simulink model "sys10m_IO"  (Simulink 8.7)
settings: Solver=ode3  StartTime=0.0  StopTime=10  FixedStep=1e-2  MaxStep=1e-2  RelTol=1e-5
values from neighbouring files (symbols this model uses):
  D = 0*D    [initDyn.m]
  event = [0 1 1.10 10 ... (first row only)    [initDyn.m]
  fYred = fYGG-fYGL*inv(fYLL)*fYLG    [initDyn.m]
  KA = ExData(:,1)    [initDyn.m]
  M = 2*H/ws    [initDyn.m]
  m = 10    [initDyn.m]
  small_d = [ ... (first row only)    [initDyn.m]
  TA = ExData(:,2)    [initDyn.m]
  Tpd0 = GenData(:,6)    [initDyn.m]
  Tpq0 = GenData(:,7)    [initDyn.m]
  ws = 377    [initDyn.m]
  XXdpd = [Xd-Xpd]    [initDyn.m]
  XXpdq = [Xpq-Xpd]    [initDyn.m]
  XXqpq = [Xq-Xpq]    [initDyn.m]
  Yred = YGG-YGL*inv(YLL)*YLG    [initDyn.m]
  Zdq = [Rsm -Xpqm;Xpdm Rsm]    [initDyn.m]
undefined symbols (not defined in the file or in its folder): delta0, Efd0, Epd0, Epq0, Vref1
libraries: powerlib_extras x2
settings Model: Creator=hbeiran  LastModifiedBy=EBUKA
settings SolverCC: AlgebraicLoopSolver=LineSearch
settings DataIOCC: LimitDataPoints=off  SignalLoggingSaveFormat=ModelDataLogs
settings OptimizationCC: DefaultParameterBehavior=Inlined  BufferReuse=off  ExpressionDepthLimit=2147483647
settings DebuggingCC: AlgebraicLoopMsg=none  SolverPrmCheckMsg=warning  FcnCallInpInsideContextMsg=UseLocalSettings  StateNameClashWarn=warning  InitInArrayFormatMsg=none
settings SFSimCC: SimParseCustomCode=off
settings GRTTargetCC: CombineOutputUpdateFcns=off  GRTInterface=on

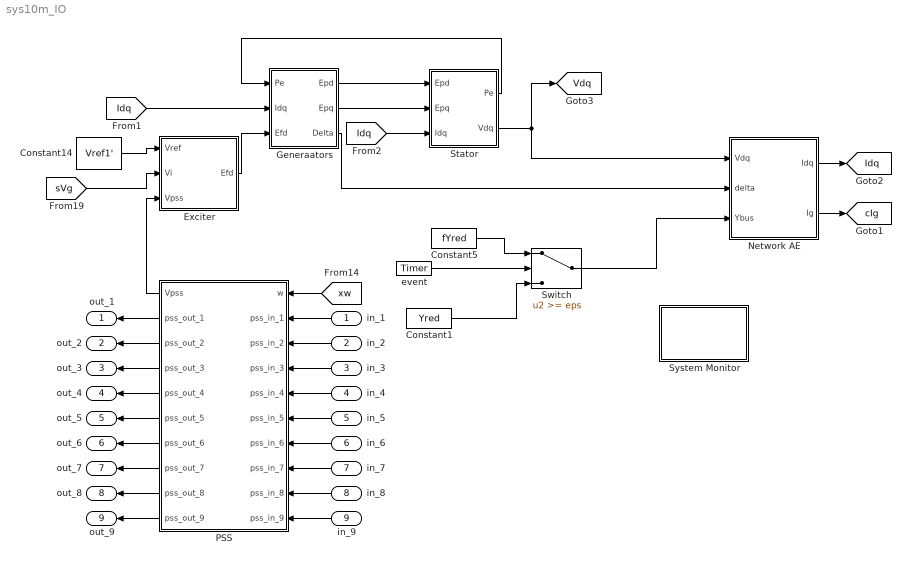
== system sys10m_IO ==
  in_1 : Inport
  in_2 : Inport  Port=2
  in_3 : Inport  Port=3
  in_4 : Inport  Port=4
  in_5 : Inport  Port=5
  in_6 : Inport  Port=6
  in_7 : Inport  Port=7
  in_8 : Inport  Port=8
  in_9 : Inport  Port=9
  Constant1 : Constant  Value=Yred  VectorParams1D=off
  Constant14 : Constant  Value=Vref1'  VectorParams1D=off
  Constant5 : Constant  Value=fYred  VectorParams1D=off
  Exciter : Subsystem
  Generaators : Subsystem
  Network AE : MATLAB Function  TreatAsAtomicUnit=on
  PSS : Subsystem
  Stator : Subsystem
  Switch : Switch  Threshold=eps
  System Monitor : Subsystem
  event : powerlib_extras/Control  Blocks/Timer  t=event(1,:)  e=event(2,:)
  out_1 : Outport
  out_2 : Outport  Port=2
  out_3 : Outport  Port=3
  out_4 : Outport  Port=4
  out_5 : Outport  Port=5
  out_6 : Outport  Port=6
  out_7 : Outport  Port=7
  out_8 : Outport  Port=8
  out_9 : Outport  Port=9
  tag scope: Idq=global, Vdq=global, cIg=global
  wires:
  Exciter/1(Efd) -> Generaators/3(Efd)
  Constant14/1 -> Exciter/1(Vref)
  Network AE/1(Idq) -> [Idq]
  event/1 -> Switch/2
  Constant5/1 -> Switch/1
  Constant1/1 -> Switch/3
  Switch/1 -> Network AE/3(Ybus)
  Generaators/3(Delta) -> Network AE/2(delta)
  Network AE/2(Ig) -> [cIg]
  Stator/2(Vdq) -> [Vdq], Network AE/1(Vdq)
  [Idq] -> Stator/3(Idq)
  Generaators/1(Epd) -> Stator/1(Epd)
  Generaators/2(Epq) -> Stator/2(Epq)
  Stator/1(Pe) -> Generaators/1(Pe)
  [sVg] -> Exciter/2(Vi)
  [Idq] -> Generaators/2(Idq)
  [xw] -> PSS/1(w)
  in_1/1 -> PSS/2(pss_in_1)
  in_2/1 -> PSS/3(pss_in_2)
  PSS/1(Vpss) -> Exciter/3(Vpss)
  PSS/2(pss_out_1) -> out_1/1
  PSS/3(pss_out_2) -> out_2/1
  in_3/1 -> PSS/4(pss_in_3)
  in_4/1 -> PSS/5(pss_in_4)
  in_5/1 -> PSS/6(pss_in_5)
  in_6/1 -> PSS/7(pss_in_6)
  in_7/1 -> PSS/8(pss_in_7)
  in_8/1 -> PSS/9(pss_in_8)
  in_9/1 -> PSS/10(pss_in_9)
  PSS/4(pss_out_3) -> out_3/1
  PSS/5(pss_out_4) -> out_4/1
  PSS/6(pss_out_5) -> out_5/1
  PSS/7(pss_out_6) -> out_6/1
  PSS/8(pss_out_7) -> out_7/1
  PSS/9(pss_out_8) -> out_8/1
  PSS/10(pss_out_9) -> out_9/1

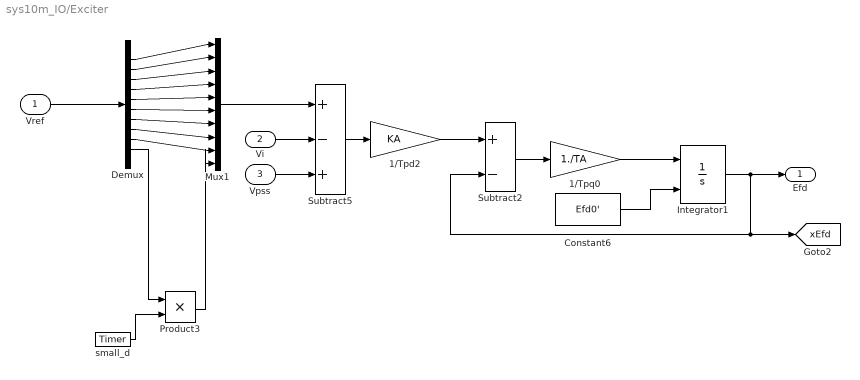
== system sys10m_IO/Exciter ==
  Vref : Inport
  Vi : Inport  Port=2
  Vpss : Inport  Port=3
  1/Tpd2 : Gain  Gain=KA
  1/Tpq0 : Gain  Gain=1./TA
  Constant6 : Constant  Value=Efd0'  VectorParams1D=off
  Demux : Demux  Outputs=10
  Integrator1 : Integrator  InitialConditionSource=external
  Mux1 : Mux  Inputs=10
  Product3 : Product  RndMeth=Zero
  Subtract2 : Sum  Inputs=+-
  Subtract5 : Sum  Inputs=+-+
  small_d : powerlib_extras/Control  Blocks/Timer  t=small_d(1,:)  e=small_d(2,:)
  Efd : Outport
  tag scope: xEfd=global
  wires:
  Constant6/1 -> Integrator1/2
  Subtract2/1 -> 1/Tpq0/1
  1/Tpq0/1 -> Integrator1/1
  Integrator1/1 -> Efd/1, Subtract2/2, [xEfd]
  Vi/1 -> Subtract5/2
  Subtract5/1 -> 1/Tpd2/1
  1/Tpd2/1 -> Subtract2/1
  Demux/1 -> Mux1/1
  Demux/2 -> Mux1/2
  small_d/1 -> Product3/2
  Mux1/1 -> Subtract5/1
  Vref/1 -> Demux/1
  Product3/1 -> Mux1/10
  Demux/10 -> Product3/1
  Demux/3 -> Mux1/3
  Demux/4 -> Mux1/4
  Demux/5 -> Mux1/5
  Demux/6 -> Mux1/6
  Demux/7 -> Mux1/7
  Demux/8 -> Mux1/8
  Demux/9 -> Mux1/9
  Vpss/1 -> Subtract5/3

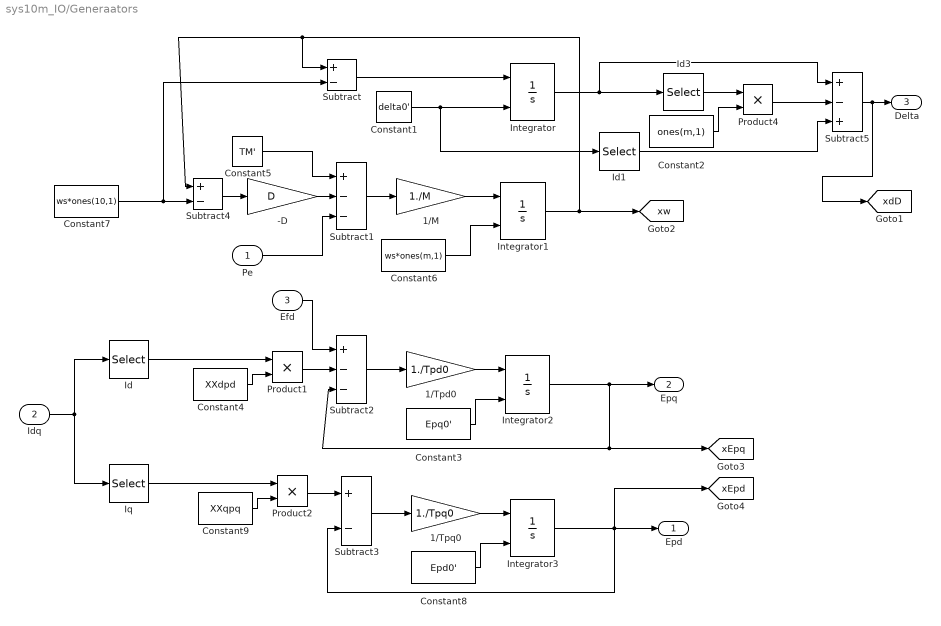
== system sys10m_IO/Generaators ==
  Pe : Inport
  Idq : Inport  Port=2
  Efd : Inport  Port=3
  -D : Gain  Gain=D
  1/M : Gain  Gain=1./M
  1/Tpd0 : Gain  Gain=1./Tpd0
  1/Tpq0 : Gain  Gain=1./Tpq0
  Constant1 : Constant  Value=delta0'  VectorParams1D=off
  Constant2 : Constant  Value=ones(m,1)  VectorParams1D=off
  Constant3 : Constant  Value=Epq0'  VectorParams1D=off
  Constant4 : Constant  Value=XXdpd  VectorParams1D=off
  Constant5 : Constant  Value=TM'  VectorParams1D=off
  Constant6 : Constant  Value=ws*ones(m,1)  VectorParams1D=off
  Constant7 : Constant  Value=ws*ones(10,1)  VectorParams1D=off
  Constant8 : Constant  Value=Epd0'  VectorParams1D=off
  Constant9 : Constant  Value=XXqpq  VectorParams1D=off
  Id : Selector  InputPortWidth=2*m  IndexOptions=Index vector (dialog)  Indices=[1:m]  OutputSizes=1
  Id1 : Selector  InputPortWidth=m  IndexOptions=Index vector (dialog)  Indices=[1]  OutputSizes=1
  Id3 : Selector  InputPortWidth=m  IndexOptions=Index vector (dialog)  Indices=[1]  OutputSizes=1
  Integrator{,1..3} (4 alike) : Integrator  InitialConditionSource=external
  Iq : Selector  InputPortWidth=2*m  IndexOptions=Index vector (dialog)  Indices=[m+1:2*m]  OutputSizes=1
  Product1 : Product  RndMeth=Zero
  Product2 : Product  RndMeth=Zero
  Product4 : Product  RndMeth=Zero
  Subtract : Sum  Inputs=+-
  Subtract1 : Sum  Inputs=+--
  Subtract2 : Sum  Inputs=+--
  Subtract3 : Sum  Inputs=+-
  Subtract4 : Sum  Inputs=+-
  Subtract5 : Sum  Inputs=+-+
  Epd : Outport
  Epq : Outport  Port=2
  Delta : Outport  Port=3
  tag scope: xEpd=global, xEpq=global, xdD=global, xw=global
  wires:
  Subtract/1 -> Integrator/1
  Constant5/1 -> Subtract1/1
  Subtract1/1 -> 1/M/1
  1/M/1 -> Integrator1/1
  Constant6/1 -> Integrator1/2
  -D/1 -> Subtract1/2
  Constant3/1 -> Integrator2/2
  Subtract2/1 -> 1/Tpd0/1
  Integrator2/1 -> Epq/1, Subtract2/3, [xEpq]
  Product1/1 -> Subtract2/2
  Constant4/1 -> Product1/2
  1/Tpd0/1 -> Integrator2/1
  Constant8/1 -> Integrator3/2
  Subtract3/1 -> 1/Tpq0/1
  Integrator3/1 -> Epd/1, [xEpd], Subtract3/2
  Constant9/1 -> Product2/2
  1/Tpq0/1 -> Integrator3/1
  Product2/1 -> Subtract3/1
  Efd/1 -> Subtract2/1
  Integrator1/1 -> [xw], Subtract/1, Subtract4/1
  Idq/1 -> Id/1, Iq/1
  Pe/1 -> Subtract1/3
  Subtract4/1 -> -D/1
  Constant7/1 -> Subtract4/2, Subtract/2
  Subtract5/1 -> Delta/1, [xdD]
  Constant1/1 -> Integrator/2, Id1/1
  Integrator/1 -> Subtract5/1, Id3/1
  Id3/1 -> Product4/1
  Constant2/1 -> Product4/2
  Product4/1 -> Subtract5/2
  Id1/1 -> Subtract5/3
  Id/1 -> Product1/1
  Iq/1 -> Product2/1

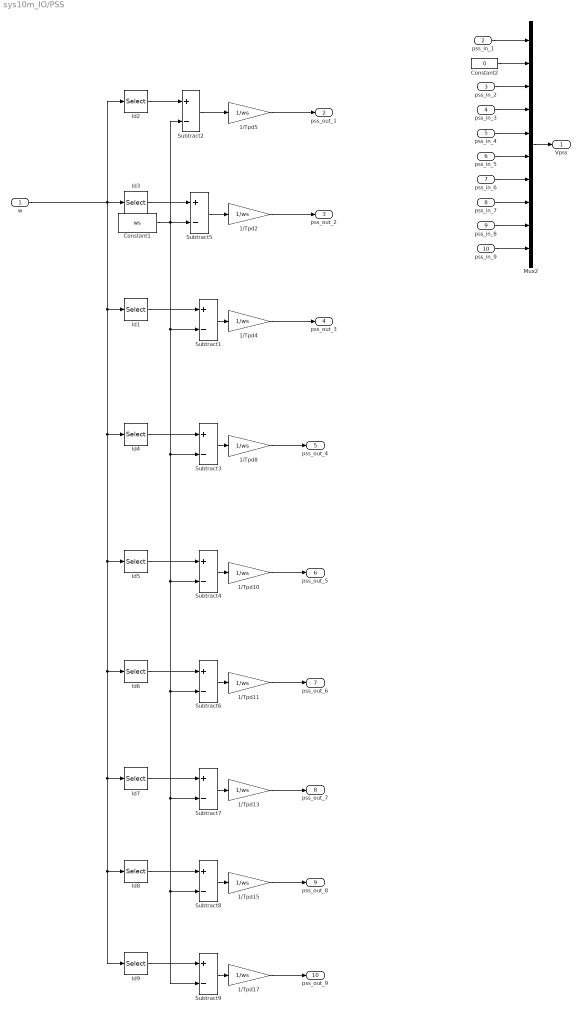
== system sys10m_IO/PSS ==
  w : Inport
  pss_in_1 : Inport  Port=2
  pss_in_2 : Inport  Port=3
  pss_in_3 : Inport  Port=4
  pss_in_4 : Inport  Port=5
  pss_in_5 : Inport  Port=6
  pss_in_6 : Inport  Port=7
  pss_in_7 : Inport  Port=8
  pss_in_8 : Inport  Port=9
  pss_in_9 : Inport  Port=10
  1/Tpd{2,4..5,8,10..11,13,15,17} (9 alike) : Gain  Gain=1/ws
  Constant1 : Constant  Value=ws  VectorParams1D=off
  Constant2 : Constant  Value=0  VectorParams1D=off
  Id1 : Selector  InputPortWidth=m  IndexOptions=Index vector (dialog)  Indices=[4]  OutputSizes=1
  Id2 : Selector  InputPortWidth=m  IndexOptions=Index vector (dialog)  Indices=[1]  OutputSizes=1
  Id3 : Selector  InputPortWidth=m  IndexOptions=Index vector (dialog)  Indices=[3]  OutputSizes=1
  Id4 : Selector  InputPortWidth=m  IndexOptions=Index vector (dialog)  Indices=[5]  OutputSizes=1
  Id5 : Selector  InputPortWidth=m  IndexOptions=Index vector (dialog)  Indices=[6]  OutputSizes=1
  Id6 : Selector  InputPortWidth=m  IndexOptions=Index vector (dialog)  Indices=[7]  OutputSizes=1
  Id7 : Selector  InputPortWidth=m  IndexOptions=Index vector (dialog)  Indices=[8]  OutputSizes=1
  Id8 : Selector  InputPortWidth=m  IndexOptions=Index vector (dialog)  Indices=[9]  OutputSizes=1
  Id9 : Selector  InputPortWidth=m  IndexOptions=Index vector (dialog)  Indices=[10]  OutputSizes=1
  Mux2 : Mux  Inputs=10
  Subtract{1..9} (9 alike) : Sum  Inputs=+-
  Vpss : Outport
  pss_out_1 : Outport  Port=2
  pss_out_2 : Outport  Port=3
  pss_out_3 : Outport  Port=4
  pss_out_4 : Outport  Port=5
  pss_out_5 : Outport  Port=6
  pss_out_6 : Outport  Port=7
  pss_out_7 : Outport  Port=8
  pss_out_8 : Outport  Port=9
  pss_out_9 : Outport  Port=10
  wires:
  Mux2/1 -> Vpss/1
  pss_in_2/1 -> Mux2/3
  pss_in_3/1 -> Mux2/4
  Constant2/1 -> Mux2/2
  pss_in_1/1 -> Mux2/1
  pss_in_4/1 -> Mux2/5
  pss_in_5/1 -> Mux2/6
  pss_in_6/1 -> Mux2/7
  pss_in_7/1 -> Mux2/8
  pss_in_8/1 -> Mux2/9
  pss_in_9/1 -> Mux2/10
  Subtract5/1 -> 1/Tpd2/1
  Id3/1 -> Subtract5/1
  Subtract1/1 -> 1/Tpd4/1
  Id1/1 -> Subtract1/1
  Id2/1 -> Subtract2/1
  Subtract2/1 -> 1/Tpd5/1
  Subtract3/1 -> 1/Tpd8/1
  Id4/1 -> Subtract3/1
  w/1 -> Id2/1, Id3/1, Id6/1, Id8/1, Id9/1, Id7/1, Id5/1, Id4/1, Id1/1
  Subtract4/1 -> 1/Tpd10/1
  Id5/1 -> Subtract4/1
  Subtract6/1 -> 1/Tpd11/1
  Id6/1 -> Subtract6/1
  Subtract7/1 -> 1/Tpd13/1
  Id7/1 -> Subtract7/1
  Subtract8/1 -> 1/Tpd15/1
  Id8/1 -> Subtract8/1
  Constant1/1 -> Subtract2/2, Subtract5/2, Subtract7/2, Subtract9/2, Subtract8/2, Subtract6/2, Subtract4/2, Subtract3/2, Subtract1/2
  Subtract9/1 -> 1/Tpd17/1
  Id9/1 -> Subtract9/1
  1/Tpd5/1 -> pss_out_1/1
  1/Tpd2/1 -> pss_out_2/1
  1/Tpd4/1 -> pss_out_3/1
  1/Tpd8/1 -> pss_out_4/1
  1/Tpd10/1 -> pss_out_5/1
  1/Tpd11/1 -> pss_out_6/1
  1/Tpd13/1 -> pss_out_7/1
  1/Tpd15/1 -> pss_out_8/1
  1/Tpd17/1 -> pss_out_9/1

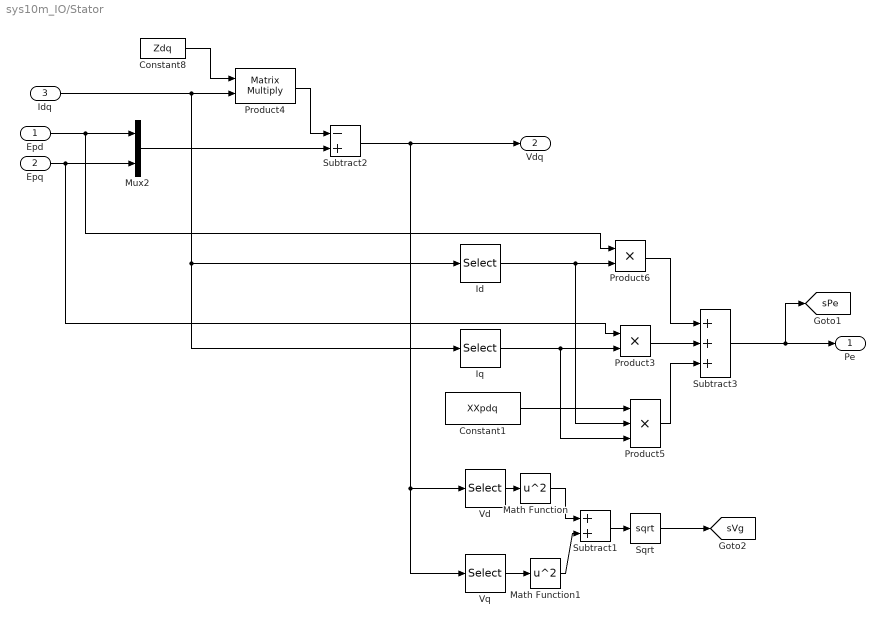
== system sys10m_IO/Stator ==
  Epd : Inport
  Epq : Inport  Port=2
  Idq : Inport  Port=3
  Constant1 : Constant  Value=XXpdq  VectorParams1D=off
  Constant8 : Constant  Value=Zdq  VectorParams1D=off
  Id : Selector  InputPortWidth=2*m  IndexOptions=Index vector (dialog)  Indices=[1:m]  OutputSizes=1
  Iq : Selector  InputPortWidth=2*m  IndexOptions=Index vector (dialog)  Indices=[m+1:2*m]  OutputSizes=1
  Math Function : Math  Operator=square  SaturateOnIntegerOverflow=on
  Math Function1 : Math  Operator=square  SaturateOnIntegerOverflow=on
  Mux2 : Mux  Inputs=2
  Product3 : Product  RndMeth=Zero
  Product4 : Product  Multiplication=Matrix(*)  RndMeth=Zero
  Product5 : Product  Inputs=3  RndMeth=Zero
  Product6 : Product  RndMeth=Zero
  Sqrt : Sqrt  SaturateOnIntegerOverflow=on
  Subtract1 : Sum
  Subtract2 : Sum  Inputs=-+
  Subtract3 : Sum  Inputs=+++
  Vd : Selector  InputPortWidth=2*m  IndexOptions=Index vector (dialog)  Indices=[1:m]  OutputSizes=1
  Vq : Selector  InputPortWidth=2*m  IndexOptions=Index vector (dialog)  Indices=[m+1:2*m]  OutputSizes=1
  Pe : Outport
  Vdq : Outport  Port=2
  tag scope: sPe=global, sVg=global
  wires:
  Constant8/1 -> Product4/1
  Epd/1 -> Mux2/1, Product6/1
  Epq/1 -> Product3/1, Mux2/2
  Iq/1 -> Product5/3, Product3/2
  Product6/1 -> Subtract3/1
  Product3/1 -> Subtract3/2
  Product5/1 -> Subtract3/3
  Constant1/1 -> Product5/1
  Subtract3/1 -> Pe/1, [sPe]
  Id/1 -> Product6/2, Product5/2
  Vd/1 -> Math Function/1
  Vq/1 -> Math Function1/1
  Math Function/1 -> Subtract1/1
  Math Function1/1 -> Subtract1/2
  Subtract1/1 -> Sqrt/1
  Sqrt/1 -> [sVg]
  Mux2/1 -> Subtract2/2
  Product4/1 -> Subtract2/1
  Subtract2/1 -> Vdq/1, Vq/1, Vd/1
  Idq/1 -> Id/1, Iq/1, Product4/2

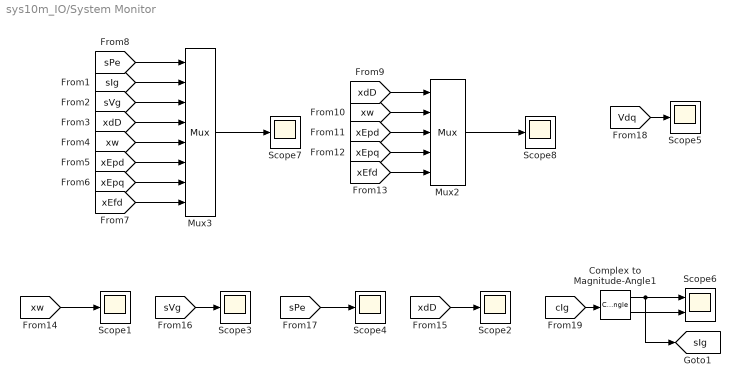
== system sys10m_IO/System Monitor ==
  Complex to Magnitude-Angle1 : ComplexToMagnitudeAngle
  Mux2 : Mux  Inputs=5
  Mux3 : Mux  Inputs=8
  Scope{1..5,7..8} (7 alike) : Scope
  Scope6 : Scope  NumInputPorts=2
  tag scope: sIg=global
  wires:
  Mux3/1 -> Scope7/1
  [sPe] -> Mux3/1
  [sIg] -> Mux3/2
  [sVg] -> Mux3/3
  [xdD] -> Mux3/4
  [xw] -> Mux3/5
  [xEpd] -> Mux3/6
  [xEpq] -> Mux3/7
  [xEfd] -> Mux3/8
  [xw] -> Mux2/2
  [xEpd] -> Mux2/3
  [xEpq] -> Mux2/4
  [xEfd] -> Mux2/5
  [xdD] -> Mux2/1
  Mux2/1 -> Scope8/1
  [xw] -> Scope1/1
  [xdD] -> Scope2/1
  [sVg] -> Scope3/1
  [sPe] -> Scope4/1
  Complex to Magnitude-Angle1/1 -> Scope6/1, [sIg]
  Complex to Magnitude-Angle1/2 -> Scope6/2
  [cIg] -> Complex to Magnitude-Angle1/1
  [Vdq] -> Scope5/1

== matlab function Network AE ==
  data: Vdq input double; Idq output double; delta input double; Ig output double; Ybus input double
function [Idq, Ig] = fcn(Vdq,delta,Ybus)
%#codegen
% global_var

% Idq

Tm = diag(exp(1j*(delta-pi/2)));
iTm = diag(exp(-1j*(delta-pi/2)));
% iTm = inv(Tm);
% Tm=eye(3);
Vg = Tm*(Vdq(1:10,1)+1j*Vdq(11:20,1));
% VLoad=VL(4:9,1);
% Vbus=[Vg;VLoad];


I = Ybus*Vg;
Ig=I(1:10,1);
Id=real(iTm*Ig);
Iq=imag(iTm*Ig);

Idq=[Id;Iq];
